simulink model "CL1CM2"  (R2024a)
settings: Solver=VariableStepAuto  StartTime=0.0  StopTime=10.0  RelTol=1e-3
settings Model: Creator=jeonghyun  LastModifiedBy=gluts

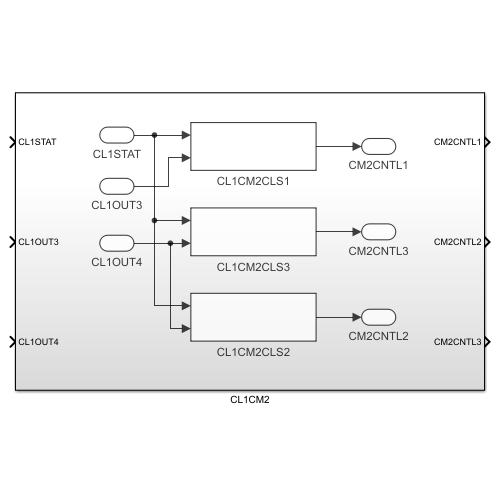
[thumbnail: Simulink's stored preview of the top-level diagram]
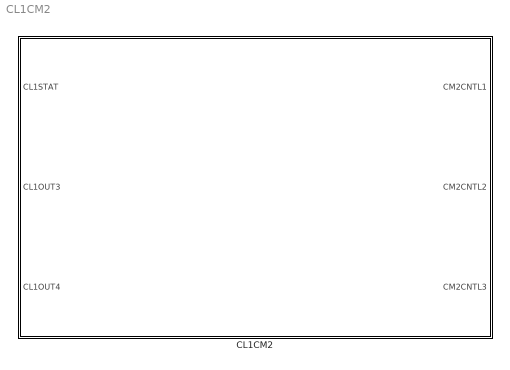
== system CL1CM2 ==
  CL1CM2 : Subsystem

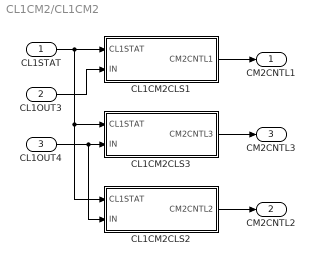
== system CL1CM2/CL1CM2 ==
  CL1STAT : Inport
  CL1OUT3 : Inport  Port=2
  CL1OUT4 : Inport  Port=3
  CL1CM2CLS1 : Subsystem
  CL1CM2CLS2 : Subsystem
  CL1CM2CLS3 : Subsystem
  CM2CNTL1 : Outport
  CM2CNTL2 : Outport  Port=2
  CM2CNTL3 : Outport  Port=3
  wires:
  CL1STAT/1 -> CL1CM2CLS3/1(CL1STAT), CL1CM2CLS2/1(CL1STAT), CL1CM2CLS1/1(CL1STAT)
  CL1CM2CLS2/1(CM2CNTL2) -> CM2CNTL2/1
  CL1CM2CLS3/1(CM2CNTL3) -> CM2CNTL3/1
  CL1OUT3/1 -> CL1CM2CLS1/2(IN)
  CL1CM2CLS1/1(CM2CNTL1) -> CM2CNTL1/1
  CL1OUT4/1 -> CL1CM2CLS2/2(IN), CL1CM2CLS3/2(IN)

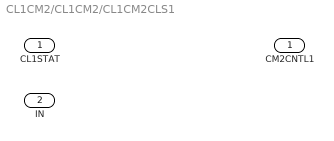
== system CL1CM2/CL1CM2/CL1CM2CLS1 ==
  CL1STAT : Inport
  IN : Inport  Port=2
  CM2CNTL1 : Outport

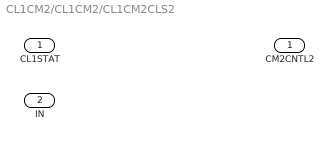
== system CL1CM2/CL1CM2/CL1CM2CLS2 ==
  CL1STAT : Inport
  IN : Inport  Port=2
  CM2CNTL2 : Outport

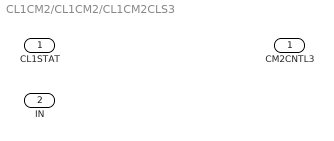
== system CL1CM2/CL1CM2/CL1CM2CLS3 ==
  CL1STAT : Inport
  IN : Inport  Port=2
  CM2CNTL3 : Outport
